simulink model "task_1_2_v01_2017b_compatible"  (R2018a)
settings: Solver=VariableStepAuto  StartTime=0.0  StopTime=1000  RelTol=1e-3
values from neighbouring files (symbols this model uses):
  faultMag = [1 0 0]    [ProblemData.m]
  faultTime = [1e6 1e6 1e6]    [ProblemData.m]
  lambda = 0.5    [ProblemData.m]
  pipeCoeff = [1 1 1]    [ProblemData.m]
  pipeCoeffNom = pipeCoeff * (1 + 0.1 * (rand(1) - 1/2))    [ProblemData.m]
  pipeCross = [5 5 5]*1e-4    [ProblemData.m]
  pipeCrossNom = pipeCross * (1 + 0.1 * (rand(1) - 1/2))    [ProblemData.m]
  pumpConst = [1.5 1.5]*1e-3    [ProblemData.m]
  seed1 = randi([1 100000])    [ProblemData.m]
  seed2 = randi([1 100000])    [ProblemData.m]
  seed3 = randi([1 100000])    [ProblemData.m]
  tankCross = [0.156 0.156 0.156]    [ProblemData.m]
  tankCrossNom = tankCross * (1 + 0.1 * (rand(1) - 1/2))    [ProblemData.m]
  tankInit = [0 2.5 5]    [ProblemData.m]
  tankInitNom = tankInit * (1 + 0.1 * (rand(1) - 1/2))    [ProblemData.m]
  tankMax = [10 10 10]    [ProblemData.m]
  tankMaxNom = tankMax * (1 + 0.1 * (rand(1) - 1/2))    [ProblemData.m]
  tankMin = [0 0 0]    [ProblemData.m]
undefined symbols (not defined in the file or in its folder): DiscIntNeverNeededParam
(part 2 of 2)

== system task_1_2_v01_2017b_compatible/3 tanks (real)/Tank2 ==
  Inflow : Inport
  Initial Level : Constant  Value=x_0
  Integrator : Integrator  InitialConditionSource=external  LimitOutput=on  UpperSaturationLimit=max_level  LowerSaturationLimit=min_level
  Tank Section : Gain  Gain=1/S  SaturateOnIntegerOverflow=on  OutDataTypeStr=Inherit: Same as input  ParamDataTypeStr=Inherit: Same as input
  Level : Outport  InitialOutput=0
  wires:
  Integrator/1 -> Level/1
  Initial Level/1 -> Integrator/2
  Tank Section/1 -> Integrator/1
  Inflow/1 -> Tank Section/1

== system task_1_2_v01_2017b_compatible/3 tanks (real)/Tank3 ==
  Inflow : Inport
  Initial Level : Constant  Value=x_0
  Integrator : Integrator  InitialConditionSource=external  LimitOutput=on  UpperSaturationLimit=max_level  LowerSaturationLimit=min_level
  Tank Section : Gain  Gain=1/S  SaturateOnIntegerOverflow=on  OutDataTypeStr=Inherit: Same as input  ParamDataTypeStr=Inherit: Same as input
  Level : Outport  InitialOutput=0
  wires:
  Integrator/1 -> Level/1
  Initial Level/1 -> Integrator/2
  Tank Section/1 -> Integrator/1
  Inflow/1 -> Tank Section/1

== system task_1_2_v01_2017b_compatible/3 tanks (real)/Valve ==
  In1 : Inport
  Enable : EnablePort  StatesWhenEnabling=reset  ShowOutputPort=on
  Product : Product  SaturateOnIntegerOverflow=on  InputSameDT=on  OutDataTypeStr=Inherit: Same as first input
  Saturation : Saturate  UpperLimit=1.0  LowerLimit=0.0
  Out1 : Outport  OutputWhenDisabled=reset  InitialOutput=0
  wires:
  Enable/1 -> Saturation/1
  Saturation/1 -> Product/1
  In1/1 -> Product/2
  Product/1 -> Out1/1

== system task_1_2_v01_2017b_compatible/3 tanks (real)/Valve1 ==
  In1 : Inport
  Enable : EnablePort  StatesWhenEnabling=reset  ShowOutputPort=on
  Product : Product  SaturateOnIntegerOverflow=on  InputSameDT=on  OutDataTypeStr=Inherit: Same as first input
  Saturation : Saturate  UpperLimit=1.0  LowerLimit=0.0
  Out1 : Outport  OutputWhenDisabled=reset  InitialOutput=0
  wires:
  Enable/1 -> Saturation/1
  Saturation/1 -> Product/1
  In1/1 -> Product/2
  Product/1 -> Out1/1

== system task_1_2_v01_2017b_compatible/3 tanks (real)/Valve2 ==
  In1 : Inport
  Enable : EnablePort  StatesWhenEnabling=reset  ShowOutputPort=on
  Product : Product  SaturateOnIntegerOverflow=on  InputSameDT=on  OutDataTypeStr=Inherit: Same as first input
  Saturation : Saturate  UpperLimit=1.0  LowerLimit=0.0
  Out1 : Outport  OutputWhenDisabled=reset  InitialOutput=0
  wires:
  Enable/1 -> Saturation/1
  Saturation/1 -> Product/1
  In1/1 -> Product/2
  Product/1 -> Out1/1
